simulink model "example6_dcmotor_sim"  (R2021b)
settings: Solver=VariableStepAuto  StartTime=0.0  StopTime=20  RelTol=1e-3
values from neighbouring files (symbols this model uses):
  J = 0.02    [example6_dcmotor.m]
  K = acker(A,B,p)    [example4_pp.m]    (also in example6_dcmotor.m = 5)
  Kb = 0.1    [example6_dcmotor.m]
  Kf = 0.2    [example6_dcmotor.m]
  Kff = 1/dcgain(dcm(1))    [example6_dcmotor.m]
  Km = 0.1    [example6_dcmotor.m]
  L = 0.5    [example6_dcmotor.m]
  R = 2.0    (= 2)    [example6_dcmotor.m]
undefined symbols (not defined in the file or in its folder): sigbuilder_block
settings Model: Creator=junmoon  LastModifiedBy=user

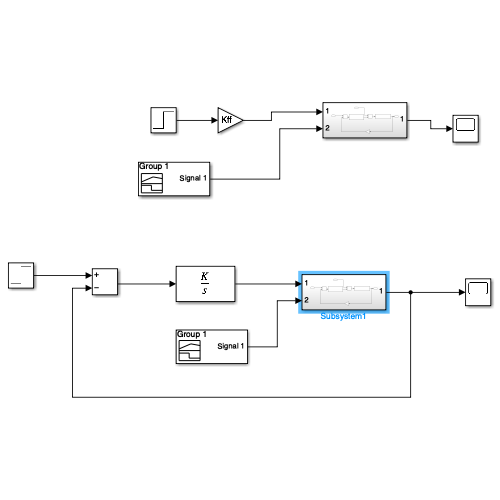
[thumbnail: Simulink's stored preview of the top-level diagram]
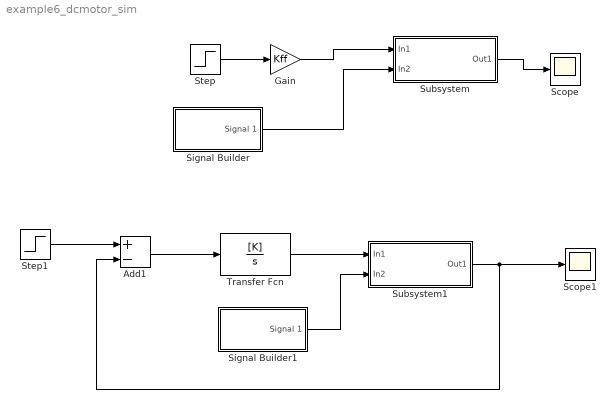
== system example6_dcmotor_sim ==
  Add1 : Sum  Inputs=+-
  Gain : Gain  Gain=Kff
  Scope : Scope
  Scope1 : Scope
  Signal Builder : Subsystem  Tag=STV Subsys  LoadFcn=sigbuilder_block('load');  StartFcn=sigbuilder_block('start');  StopFcn=sigbuilder_block('stop');  ClipboardFcn=sigbuilder_block('clipboard');  mask(Sigbuilder block){tuvar=[0:10]}
      mask help: Simulink:masks:SigbuilderBlock_MD
      mask init:
      | if ~strcmp(get_param(bdroot(gcbh),'SimulationStatus'),'stopped') tuvar = sigbuilder_block('maskInit'); end
      settings: CopyFcn=sigbuilder_block('copy');  DeleteFcn=sigbuilder_block('delete');  ModelCloseFcn=sigbuilder_block('modelClose');  PreSaveFcn=sigbuilder_block('preSave');  PauseFcn=sigbuilder_block('pause');  ContinueFcn=sigbuilder_block('continue');  NameChangeFcn=sigbuilder_block('namechange');  OpenFcn=sigbuilder_block('open',[437.6 199.2 851.4 400 ]);  CloseFcn=sigbuilder_block('close');
      mask Display: plot(0, 0, 100, 100,[2, 2, 32, 32, 2], [68, 8, 8, 68, 68],[32, 2], [38, 38], [32, 19, 2],[53, 60, 44], [32, 17, 17, 2],[16, 16, 31, 31]);txt = getActiveGroup(gcbh);text(2, 100, txt,'verticalAlignment', 'top');
  Signal Builder1 : Subsystem  Tag=STV Subsys  LoadFcn=sigbuilder_block('load');  StartFcn=sigbuilder_block('start');  StopFcn=sigbuilder_block('stop');  ClipboardFcn=sigbuilder_block('clipboard');  mask(Sigbuilder block){tuvar=[0:10]}
      mask help: Simulink:masks:SigbuilderBlock_MD
      mask init:
      | if ~strcmp(get_param(bdroot(gcbh),'SimulationStatus'),'stopped') tuvar = sigbuilder_block('maskInit'); end
      settings: CopyFcn=sigbuilder_block('copy');  DeleteFcn=sigbuilder_block('delete');  ModelCloseFcn=sigbuilder_block('modelClose');  PreSaveFcn=sigbuilder_block('preSave');  PauseFcn=sigbuilder_block('pause');  ContinueFcn=sigbuilder_block('continue');  NameChangeFcn=sigbuilder_block('namechange');  OpenFcn=sigbuilder_block('open',[437.6 199.2 851.4 400 ]);  CloseFcn=sigbuilder_block('close');
      mask Display: plot(0, 0, 100, 100,[2, 2, 32, 32, 2], [68, 8, 8, 68, 68],[32, 2], [38, 38], [32, 19, 2],[53, 60, 44], [32, 17, 17, 2],[16, 16, 31, 31]);txt = getActiveGroup(gcbh);text(2, 100, txt,'verticalAlignment', 'top');
  Step : Step  Time=0  SampleTime=0
  Step1 : Step  Time=0  SampleTime=0
  Subsystem : Subsystem
  Subsystem1 : Subsystem
  Transfer Fcn : TransferFcn  Numerator=[K]  Denominator=[1 0]
  wires:
  Gain/1 -> Subsystem/1(In1)
  Step/1 -> Gain/1
  Subsystem/1(Out1) -> Scope/1
  Signal Builder/1(Signal 1) -> Subsystem/2(In2)
  Add1/1 -> Transfer Fcn/1
  Subsystem1/1(Out1) -> Scope1/1, Add1/2
  Step1/1 -> Add1/1
  Signal Builder1/1(Signal 1) -> Subsystem1/2(In2)
  Transfer Fcn/1 -> Subsystem1/1(In1)

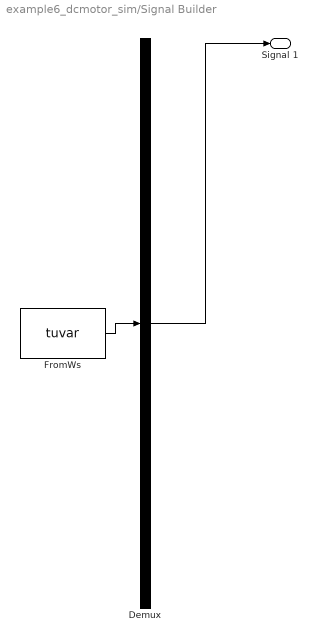
== system example6_dcmotor_sim/Signal Builder ==
  Demux : Demux  Tag=STV Demux  Outputs=1
      settings: DisplayOption=none
  FromWs : FromWorkspace  Tag=STV FromWs  VariableName=tuvar
      SigBuilderData=|
      | common.afterFinalStr = 'Extrapolate'
      | common.sampleTime = 0
      | dataSet.timeRange = [0 20]
      | dataSet.name = 'Group 1'
      | sbobj.Groups.Name = 'Group 1'
      | sbobj.Groups.Signals.Name = 'Signal 1'
      | sbobj.Groups.Signals.XData = [0 5 5 10 10 20]
      | sbobj.Groups.Signals.YData = [0 0 -0.102 -0.102 0 0]
      | sbobj.Groups.TimeRange = [0 20]
  Signal 1 : Outport  Tag=STV Outport
  wires:
  Demux/1 -> Signal 1/1
  FromWs/1 -> Demux/1

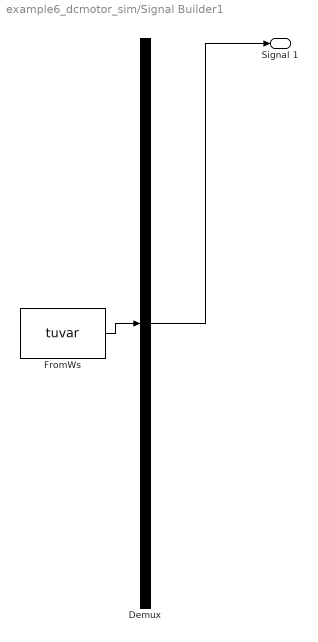
== system example6_dcmotor_sim/Signal Builder1 ==
  Demux : Demux  Tag=STV Demux  Outputs=1
      settings: DisplayOption=none
  FromWs : FromWorkspace  Tag=STV FromWs  VariableName=tuvar
      SigBuilderData=|
      | common.afterFinalStr = 'Extrapolate'
      | common.sampleTime = 0
      | dataSet.timeRange = [0 20]
      | dataSet.name = 'Group 1'
      | sbobj.Groups.Name = 'Group 1'
      | sbobj.Groups.Signals.Name = 'Signal 1'
      | sbobj.Groups.Signals.XData = [0 5 5 10 10 20]
      | sbobj.Groups.Signals.YData = [0 0 -0.102 -0.102 0 0]
      | sbobj.Groups.TimeRange = [0 20]
  Signal 1 : Outport  Tag=STV Outport
  wires:
  Demux/1 -> Signal 1/1
  FromWs/1 -> Demux/1

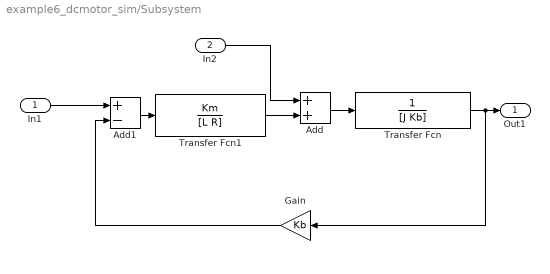
== system example6_dcmotor_sim/Subsystem ==
  In1 : Inport
  In2 : Inport  Port=2
  Add : Sum
  Add1 : Sum  Inputs=+-
  Gain : Gain  Gain=Kb
  Transfer Fcn : TransferFcn  Denominator=[J Kb]
  Transfer Fcn1 : TransferFcn  Numerator=Km  Denominator=[L R]
  Out1 : Outport
  wires:
  Transfer Fcn1/1 -> Add/2
  Add/1 -> Transfer Fcn/1
  In2/1 -> Add/1
  Add1/1 -> Transfer Fcn1/1
  In1/1 -> Add1/1
  Transfer Fcn/1 -> Gain/1, Out1/1
  Gain/1 -> Add1/2

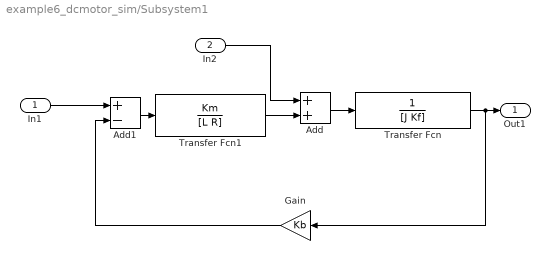
== system example6_dcmotor_sim/Subsystem1 ==
  In1 : Inport
  In2 : Inport  Port=2
  Add : Sum
  Add1 : Sum  Inputs=+-
  Gain : Gain  Gain=Kb
  Transfer Fcn : TransferFcn  Denominator=[J Kf]
  Transfer Fcn1 : TransferFcn  Numerator=Km  Denominator=[L R]
  Out1 : Outport
  wires:
  Transfer Fcn1/1 -> Add/2
  Add/1 -> Transfer Fcn/1
  In2/1 -> Add/1
  Add1/1 -> Transfer Fcn1/1
  In1/1 -> Add1/1
  Transfer Fcn/1 -> Gain/1, Out1/1
  Gain/1 -> Add1/2
